simulink model "c62e6e98"  (R2018a)
settings: Solver=ode45  StartTime=0.0  StopTime=0.5  MaxStep=1e-4  RelTol=1e-3
libraries: powerlib x10, simulink x1, powerlib_meascontrol x1
settings Model: SimulationMode=accelerator  Creator=黄永烁  LastModifiedBy=taiy
settings OptimizationCC: EfficientMapNaN2IntZero=off
settings HardwareCC: TargetBitPerPointer=64  TargetBitPerSizeT=64  TargetBitPerPtrDiffT=64  TargetLongLongMode=on  TargetIntDivRoundTo=Zero  TargetEndianess=LittleEndian  TargetWordSize=64  TargetHWDeviceType=MATLAB Host  ProdEqTarget=off
settings CodeAppCC: MaxIdLength=128
settings GRTTargetCC: TargetLangStandard=C89/C90 (ANSI)  CombineOutputUpdateFcns=off  GRTInterface=on
settings SimscapeCC: SimscapeNormalizeSystem=off

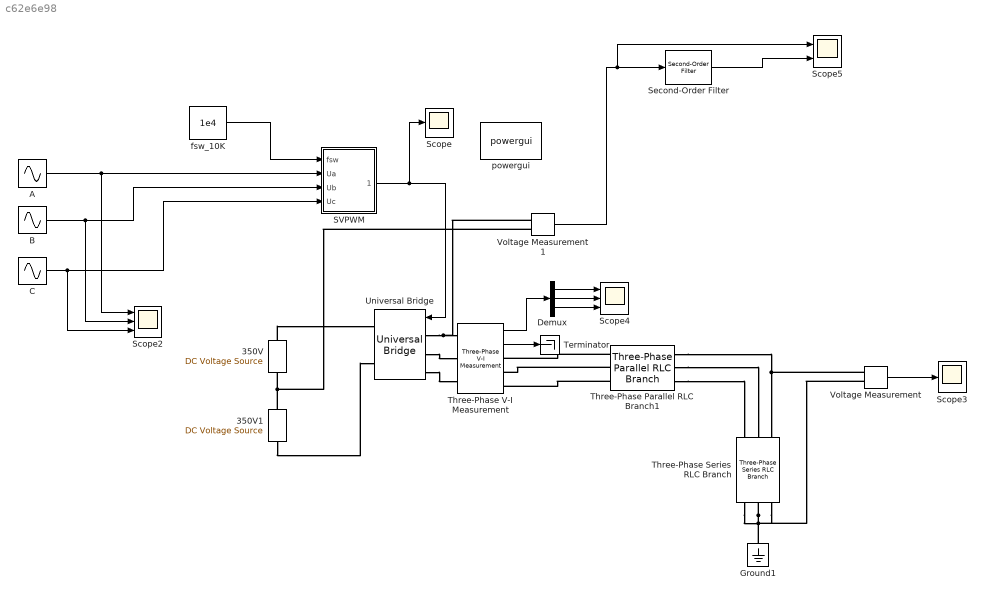
== system c62e6e98 ==
  350V : powerlib/Electrical Sources/DC Voltage Source  Amplitude=350  Measurements=None
  350V1 : powerlib/Electrical Sources/DC Voltage Source  Amplitude=350  Measurements=None
  A : Sin  Amplitude=311  Frequency=100*pi  SampleTime=0
  B : Sin  Amplitude=311  Frequency=100*pi  Phase=-2*pi/3  SampleTime=0
  C : Sin  Amplitude=311  Frequency=100*pi  Phase=2*pi/3  SampleTime=0
  Demux : Demux  Outputs=3
  Ground1 : powerlib/Elements/Ground  LConnTagsString=a
  SVPWM : Subsystem
  Scope : Scope
  Scope2 : Scope  NumInputPorts=3
  Scope3 : Scope
  Scope4 : Scope  NumInputPorts=3
  Scope5 : Scope  NumInputPorts=2
  Second-Order Filter : powerlib_meascontrol/Filters/Second-Order Filter  FilterType=Lowpass  Fo=600  Zeta=0.707  Ts=0  Initialize=on  Vac_Init="[0,  0,  50]"  Vdc_Init=0  PlotResponse=off  FreqRange=[0, 500, 1]
      settings: SourceProductName=Simscape Power Systems  SourceProductBaseCode=PS
  Terminator : Terminator
  Three-Phase Parallel RLC Branch1 : powerlib/Elements/Three-Phase Parallel RLC Branch  LConnTagsString=A|B|C  RConnTagsString=A|B|C  BranchType=R  Resistance=10000  Inductance=20e-3  Capacitance=1e-6  Measurements=None
      settings: SourceProductName=Simscape Power Systems  SourceProductBaseCode=PS
  Three-Phase Series RLC Branch : powerlib/Elements/Three-Phase Series RLC Branch  LConnTagsString=A|B|C  RConnTagsString=A|B|C  BranchType=C  Resistance=15  Inductance=1e-3  Capacitance=1e-7  Measurements=None
  Three-Phase V-I Measurement : powerlib/Measurements/Three-Phase V-I Measurement  VoltageMeasurement=phase-to-ground  SetLabelV=off  LabelV=Vabc  Vpu=off  VpuLL=off  CurrentMeasurement=yes  SetLabelI=off  LabelI=Iabc  Ipu=off  Pbase=3000  Vbase=381  OutputType=Complex  PhasorSimulation=off  PSBequivalent=0
  Universal Bridge : powerlib/Power Electronics/Universal Bridge  Arms=3  SnubberResistance=1e5  SnubberCapacitance=inf  Device=IGBT / Diodes  Ron=1e-3  Lon=0  ForwardVoltages="[  0  0  ]"  ForwardVoltage=0  GTOparameters=[ 10e-6 , 20e-6 ]  IGBTparameters=[ 1e-6 , 2e-6 ]  Measurements=None  Measurements_2=None  converterType=Rectifier
  Voltage Measurement : powerlib/Measurements/Voltage Measurement  PhasorSimulation=off  OutputType=Complex  PSBequivalent=0
  Voltage Measurement1 : powerlib/Measurements/Voltage Measurement  PhasorSimulation=off  OutputType=Complex  PSBequivalent=0
  fsw_10K : Constant  Value=1e4
  powergui : powerlib/powergui  Priority=1  SimulationMode=Discrete  SampleTime=1e-6  frequency=60  Iterations=50  frequencyindice=0  Pbase=100e6  ErrMax=1e-4  UnitsV=kV  UnitsW=MW  buscounter=0  FunctionMessages=off  echomessages=off  EnableUseOfTLC=off  CurrentSourceSwitches=off  DisableSnubberDevices=off  DisableRonSwitches=off  DisableVfSwitches=off  DisplayEquations=off  SolverType=Tustin/Backward Euler (TBE)  Interpol=off  ExternalGateDelay=off  methode=off  Ts=100  x0status=blocks  SPID=on  SwTol=0  HookPort=off  RestoreLinks=warning  ResistiveCurrentMeasurement=off  Frange=[0:2:500]  Ylog=off  Xlog=on  ShowGrid=off  save=off  variable=ZData  structure=IL1  ZoomFFT=off  StartTime=0.1  cycles=2  DisplayStyle=3  fundamental=50  FreqAxis=off  MaxFrequency=1.5e4  frequencyindicesteady=1  RmsSteady=1  display=off
  wires:
  A/1 -> Scope2/1, SVPWM/2(Ua)
  C/1 -> Scope2/3, SVPWM/4(Uc)
  B/1 -> Scope2/2, SVPWM/3(Ub)
  fsw_10K/1 -> SVPWM/1(fsw)
  SVPWM/1(SVPWM) -> Scope/1, Universal Bridge/1
  Demux/2 -> Scope4/2
  Demux/1 -> Scope4/1
  Demux/3 -> Scope4/3
  Three-Phase V-I Measurement/1 -> Demux/1
  Voltage Measurement/1 -> Scope3/1
  Second-Order Filter/1 -> Scope5/2
  Voltage Measurement1/1 -> Second-Order Filter/1, Scope5/1
  Three-Phase V-I Measurement/2 -> Terminator/1
  connections:
  Three-Phase Parallel RLC Branch1/RConn1 -- Voltage Measurement/LConn1 -- Three-Phase Series RLC Branch/LConn3
  Three-Phase Parallel RLC Branch1/RConn3 -- Three-Phase Series RLC Branch/LConn1
  Three-Phase Parallel RLC Branch1/RConn2 -- Three-Phase Series RLC Branch/LConn2
  Three-Phase Series RLC Branch/RConn2 -- Voltage Measurement/LConn2 -- Three-Phase Series RLC Branch/RConn3 -- Ground1/LConn1 -- Three-Phase Series RLC Branch/RConn1
  350V/RConn1 -- Universal Bridge/RConn1
  Universal Bridge/LConn1 -- Voltage Measurement1/LConn1 -- Three-Phase V-I Measurement/LConn1
  Universal Bridge/LConn2 -- Three-Phase V-I Measurement/LConn2
  Three-Phase Parallel RLC Branch1/LConn1 -- Three-Phase V-I Measurement/RConn1
  Universal Bridge/LConn3 -- Three-Phase V-I Measurement/LConn3
  Three-Phase Parallel RLC Branch1/LConn3 -- Three-Phase V-I Measurement/RConn3
  Three-Phase Parallel RLC Branch1/LConn2 -- Three-Phase V-I Measurement/RConn2
  350V1/RConn1 -- Voltage Measurement1/LConn2 -- 350V/LConn1
  350V1/LConn1 -- Universal Bridge/RConn2

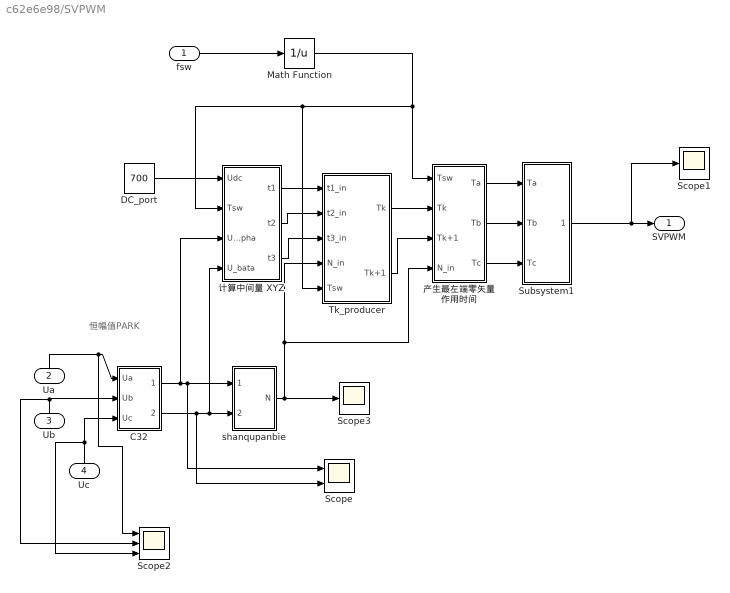
== system c62e6e98/SVPWM ==
  note: 恒幅值PARK
  fsw : Inport
  Ua : Inport  Port=2
  Ub : Inport  Port=3
  Uc : Inport  Port=4
  C32 : Subsystem
  DC_port : Constant  Value=700
  Math Function : Math  Operator=reciprocal  SaturateOnIntegerOverflow=on
  Scope : Scope  NumInputPorts=2
  Scope1 : Scope
  Scope2 : Scope  NumInputPorts=3
  Scope3 : Scope
  Subsystem1 : Subsystem
  Tk_producer : Subsystem
  shanqupanbie : Subsystem
  产生最左端零矢量 作用时间 : Subsystem
  计算中间量 XYZ : Subsystem
  SVPWM : Outport
  wires:
  Uc/1 -> Scope2/3, C32/3(Uc)
  Ua/1 -> Scope2/1, C32/1(Ua)
  Ub/1 -> Scope2/2, C32/2(Ub)
  Tk_producer/2(Tk+1) -> 产生最左端零矢量 作用时间/3(Tk+1)
  计算中间量 XYZ/2(t2) -> Tk_producer/2(t2_in)
  产生最左端零矢量 作用时间/2(Tb) -> Subsystem1/2(Tb)
  C32/2(U_b) -> Scope/2, shanqupanbie/2(bata), 计算中间量 XYZ/4(U_bata)
  产生最左端零矢量 作用时间/1(Ta) -> Subsystem1/1(Ta)
  产生最左端零矢量 作用时间/3(Tc) -> Subsystem1/3(Tc)
  shanqupanbie/1(N) -> Tk_producer/4(N_in), 产生最左端零矢量 作用时间/4(N_in), Scope3/1
  C32/1(U_a) -> Scope/1, shanqupanbie/1(alpha), 计算中间量 XYZ/3(U_alpha)
  DC_port/1 -> 计算中间量 XYZ/1(Udc)
  计算中间量 XYZ/3(t3) -> Tk_producer/3(t3_in)
  Subsystem1/1(Out1) -> Scope1/1, SVPWM/1
  Tk_producer/1(Tk) -> 产生最左端零矢量 作用时间/2(Tk)
  计算中间量 XYZ/1(t1) -> Tk_producer/1(t1_in)
  fsw/1 -> Math Function/1
  Math Function/1 -> Tk_producer/5(Tsw), 计算中间量 XYZ/2(Tsw), 产生最左端零矢量 作用时间/1(Tsw)

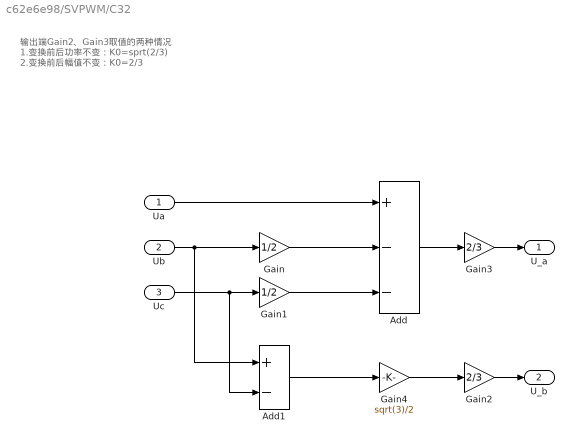
== system c62e6e98/SVPWM/C32 ==
  note: 输出端Gain2、Gain3取值的两种情况
      | 1.变换前后功率不变：K0=sprt(2/3)
      | 2.变换前后幅值不变：K0=2/3
  Ua : Inport
  Ub : Inport  Port=2
  Uc : Inport  Port=3
  Add : Sum  Inputs=+--
  Add1 : Sum  Inputs=+-
  Gain : Gain  Gain=1/2
  Gain1 : Gain  Gain=1/2
  Gain2 : Gain  Gain=2/3
  Gain3 : Gain  Gain=2/3
  Gain4 : Gain  Gain=sqrt(3)/2
  U_a : Outport
  U_b : Outport  Port=2
  wires:
  Add/1 -> Gain3/1
  Gain/1 -> Add/2
  Gain1/1 -> Add/3
  Uc/1 -> Add1/2, Gain1/1
  Ub/1 -> Add1/1, Gain/1
  Ua/1 -> Add/1
  Gain3/1 -> U_a/1
  Gain2/1 -> U_b/1
  Add1/1 -> Gain4/1
  Gain4/1 -> Gain2/1

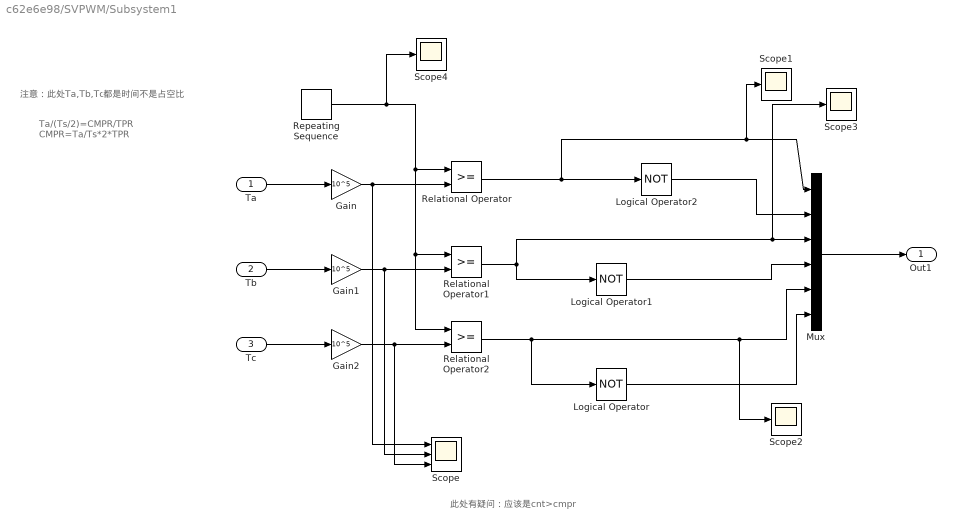
== system c62e6e98/SVPWM/Subsystem1 ==
  note: Ta/(Ts/2)=CMPR/TPR
      | CMPR=Ta/Ts*2*TPR
  note: 注意：此处Ta,Tb,Tc都是时间不是占空比
  note: 此处有疑问：应该是cnt>cmpr
  Ta : Inport
  Tb : Inport  Port=2
  Tc : Inport  Port=3
  Gain : Gain  Gain=10^5
  Gain1 : Gain  Gain=10^5
  Gain2 : Gain  Gain=10^5
  Logical Operator : Logic  Operator=NOT  AllPortsSameDT=off  OutDataTypeStr=boolean
  Logical Operator1 : Logic  Operator=NOT  AllPortsSameDT=off  OutDataTypeStr=boolean
  Logical Operator2 : Logic  Operator=NOT  AllPortsSameDT=off  OutDataTypeStr=boolean
  Mux : Mux  Inputs=6
  Relational Operator : RelationalOperator  OutDataTypeStr=boolean  RndMeth=Nearest
  Relational Operator1 : RelationalOperator  OutDataTypeStr=boolean  RndMeth=Nearest
  Relational Operator2 : RelationalOperator  OutDataTypeStr=boolean  RndMeth=Nearest
  Repeating Sequence : simulink/Sources/Repeating Sequence  rep_seq_t=[0 1/20000 1/10000]  rep_seq_y=[0 5 0]
  Scope : Scope  NumInputPorts=3
  Scope{1..4} (4 alike) : Scope
  Out1 : Outport
  wires:
  Mux/1 -> Out1/1
  Logical Operator2/1 -> Mux/2
  Logical Operator1/1 -> Mux/4
  Logical Operator/1 -> Mux/6
  Relational Operator/1 -> Logical Operator2/1, Scope1/1, Mux/1
  Relational Operator1/1 -> Logical Operator1/1, Scope3/1, Mux/3
  Relational Operator2/1 -> Logical Operator/1, Scope2/1, Mux/5
  Ta/1 -> Gain/1
  Tb/1 -> Gain1/1
  Tc/1 -> Gain2/1
  Gain/1 -> Relational Operator/2, Scope/1
  Gain1/1 -> Relational Operator1/2, Scope/2
  Gain2/1 -> Relational Operator2/2, Scope/3
  Repeating Sequence/1 -> Scope4/1, Relational Operator/1, Relational Operator1/1, Relational Operator2/1

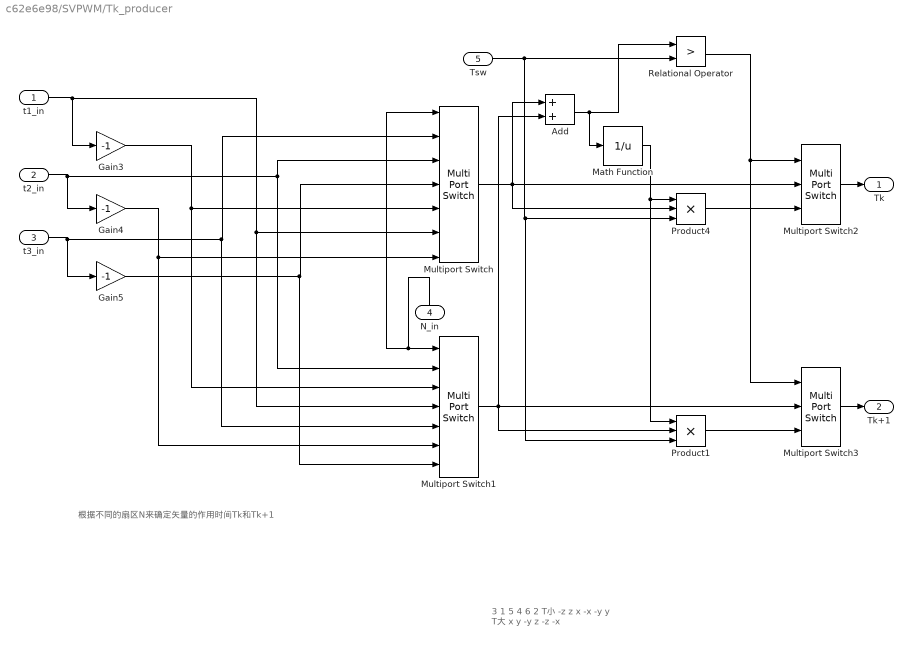
== system c62e6e98/SVPWM/Tk_producer ==
  note: 根据不同的扇区N来确定矢量的作用时间Tk和Tk+1
  note: 3  1  5  4  6  2
      | T小  -z  z  x  -x -y  y
      | T大   x  y -y   z -z -x
  t1_in : Inport
  t2_in : Inport  Port=2
  t3_in : Inport  Port=3
  N_in : Inport  Port=4
  Tsw : Inport  Port=5
  Add : Sum
  Gain3 : Gain  Gain=-1
  Gain4 : Gain  Gain=-1
  Gain5 : Gain  Gain=-1
  Math Function : Math  Operator=reciprocal  SaturateOnIntegerOverflow=on
  Multiport Switch : MultiPortSwitch  Inputs=6
  Multiport Switch1 : MultiPortSwitch  Inputs=6
  Multiport Switch2 : MultiPortSwitch  DataPortOrder=Zero-based contiguous  Inputs=2  zeroidx=on
  Multiport Switch3 : MultiPortSwitch  DataPortOrder=Zero-based contiguous  Inputs=2  zeroidx=on
  Product1 : Product  Inputs=3  RndMeth=Zero
  Product4 : Product  Inputs=3  RndMeth=Zero
  Relational Operator : RelationalOperator  Operator=>  OutDataTypeStr=boolean  RndMeth=Nearest
  Tk : Outport
  Tk+1 : Outport  Port=2
  wires:
  N_in/1 -> Multiport Switch1/1, Multiport Switch/1
  t2_in/1 -> Multiport Switch1/2, Multiport Switch/3, Gain4/1
  t3_in/1 -> Multiport Switch1/5, Multiport Switch/2, Gain5/1
  t1_in/1 -> Multiport Switch1/4, Multiport Switch/6, Gain3/1
  Multiport Switch/1 -> Product4/2, Multiport Switch2/2, Add/1
  Multiport Switch1/1 -> Product1/2, Multiport Switch3/2, Add/2
  Relational Operator/1 -> Multiport Switch3/1, Multiport Switch2/1
  Add/1 -> Math Function/1, Relational Operator/1
  Tsw/1 -> Product1/3, Product4/3, Relational Operator/2
  Multiport Switch2/1 -> Tk/1
  Multiport Switch3/1 -> Tk+1/1
  Math Function/1 -> Product1/1, Product4/1
  Product4/1 -> Multiport Switch2/3
  Product1/1 -> Multiport Switch3/3
  Gain3/1 -> Multiport Switch1/3, Multiport Switch/5
  Gain4/1 -> Multiport Switch1/6, Multiport Switch/7
  Gain5/1 -> Multiport Switch1/7, Multiport Switch/4

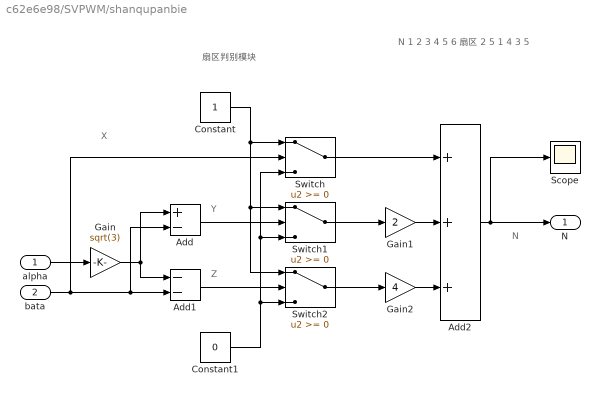
== system c62e6e98/SVPWM/shanqupanbie ==
  note: N
  note: N 1 2 3 4 5 6
      | 扇区 2 5 1 4 3 5
  note: 扇区判别模块
  note: Z
  note: Y
  note: X
  alpha : Inport
  bata : Inport  Port=2
  Add : Sum  Inputs=+-
  Add1 : Sum  Inputs=--
  Add2 : Sum  Inputs=+++
  Constant : Constant
  Constant1 : Constant  Value=0
  Gain : Gain  Gain=sqrt(3)
  Gain1 : Gain  Gain=2
  Gain2 : Gain  Gain=4
  Scope : Scope
  Switch : Switch
  Switch1 : Switch
  Switch2 : Switch
  N : Outport
  wires:
  Gain/1 -> Add/1, Add1/1
  bata/1 -> Switch/2, Add/2, Add1/2
  Add1/1 -> Switch2/2
  Add/1 -> Switch1/2
  Constant/1 -> Switch/1, Switch1/1, Switch2/1
  Constant1/1 -> Switch2/3, Switch1/3, Switch/3
  Switch2/1 -> Gain2/1
  Switch1/1 -> Gain1/1
  Gain2/1 -> Add2/3
  Gain1/1 -> Add2/2
  Switch/1 -> Add2/1
  Add2/1 -> Scope/1, N/1
  alpha/1 -> Gain/1

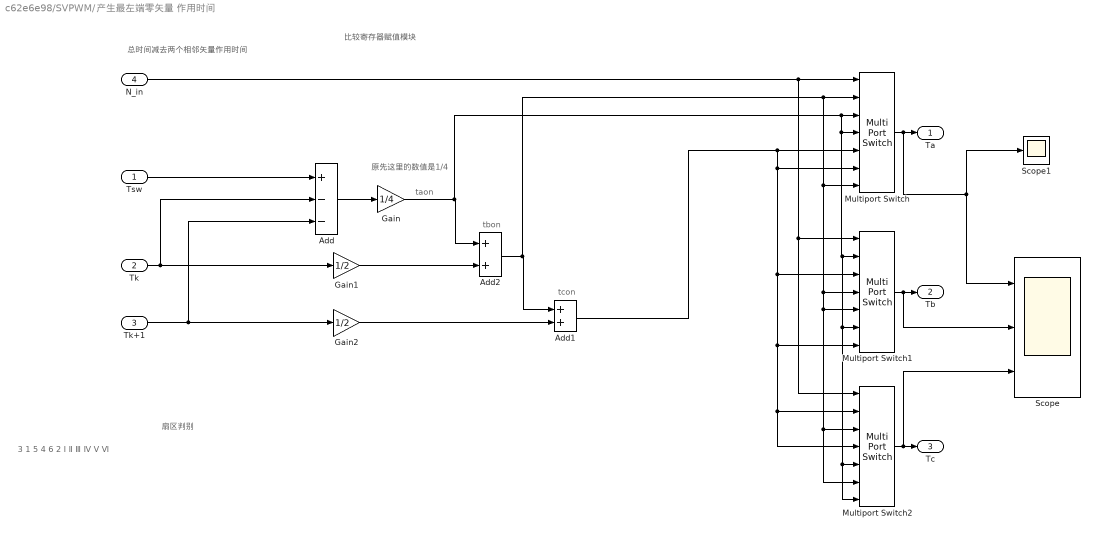
== system c62e6e98/SVPWM/产生最左端零矢量 作用时间 ==
  note: 扇区判别
  note: 3
      | 1
      | 5
      | 4
      | 6
      | 2
      |
      | Ⅰ
      | Ⅱ
      | Ⅲ
      | Ⅳ
      | Ⅴ
      | Ⅵ
  note: 原先这里的数值是1/4
  note: tcon
  note: tbon
  note: taon
  note: 比较寄存器赋值模块
  note: 总时间减去两个相邻矢量作用时间
  Tsw : Inport
  Tk : Inport  Port=2
  Tk+1 : Inport  Port=3
  N_in : Inport  Port=4
  Add : Sum  Inputs=+--
  Add1 : Sum
  Add2 : Sum
  Gain : Gain  Gain=1/4
  Gain1 : Gain  Gain=1/2
  Gain2 : Gain  Gain=1/2
  Multiport Switch : MultiPortSwitch  Inputs=6
  Multiport Switch1 : MultiPortSwitch  Inputs=6
  Multiport Switch2 : MultiPortSwitch  Inputs=6
  Scope : Scope  NumInputPorts=3
  Scope1 : Scope
  Ta : Outport
  Tb : Outport  Port=2
  Tc : Outport  Port=3
  wires:
  Add/1 -> Gain/1
  Gain/1 -> Multiport Switch2/7, Multiport Switch2/5, Multiport Switch1/6, Multiport Switch1/2, Multiport Switch/4, Multiport Switch/3, Add2/1
  Gain1/1 -> Add2/2
  Gain2/1 -> Add1/2
  Add2/1 -> Multiport Switch2/6, Multiport Switch2/3, Multiport Switch1/5, Multiport Switch1/4, Multiport Switch/7, Multiport Switch/2, Add1/1
  Tsw/1 -> Add/1
  Multiport Switch/1 -> Ta/1, Scope1/1, Scope/1
  Multiport Switch1/1 -> Tb/1, Scope/2
  Multiport Switch2/1 -> Tc/1, Scope/3
  N_in/1 -> Multiport Switch2/1, Multiport Switch1/1, Multiport Switch/1
  Tk/1 -> Add/2, Gain1/1
  Tk+1/1 -> Add/3, Gain2/1
  Add1/1 -> Multiport Switch2/4, Multiport Switch2/2, Multiport Switch1/7, Multiport Switch1/3, Multiport Switch/6, Multiport Switch/5

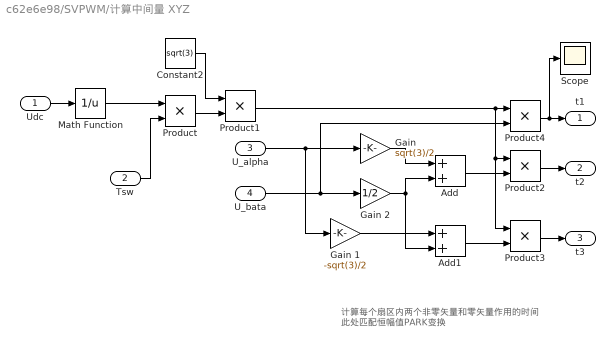
== system c62e6e98/SVPWM/计算中间量 XYZ ==
  note: 计算每个扇区内两个非零矢量和零矢量作用的时间
      |
      |
      | 此处匹配恒幅值PARK变换
  Udc : Inport
  Tsw : Inport  Port=2
  U_alpha : Inport  Port=3
  U_bata : Inport  Port=4
  " Gain" : Gain  Gain=sqrt(3)/2
  Add : Sum
  Add1 : Sum
  Constant2 : Constant  Value=sqrt(3)
  Gain 1 : Gain  Gain=-sqrt(3)/2
  Gain 2 : Gain  Gain=1/2
  Math Function : Math  Operator=reciprocal  SaturateOnIntegerOverflow=on
  Product{,1..4} (5 alike) : Product  RndMeth=Zero
  Scope : Scope
  t1 : Outport
  t2 : Outport  Port=2
  t3 : Outport  Port=3
  wires:
  Math Function/1 -> Product/1
  Product/1 -> Product1/2
  Constant2/1 -> Product1/1
  " Gain"/1 -> Add/1
  Gain 1/1 -> Add1/1
  Add/1 -> Product2/2
  Product1/1 -> Product2/1, Product3/1, Product4/1
  Add1/1 -> Product3/2
  U_alpha/1 -> Gain 1/1, " Gain"/1
  Udc/1 -> Math Function/1
  Tsw/1 -> Product/2
  Product3/1 -> t3/1
  Product2/1 -> t2/1
  Gain 2/1 -> Add/2, Add1/2
  U_bata/1 -> Gain 2/1, Product4/2
  Product4/1 -> Scope/1, t1/1
